simulink model "iir_butterworth"  (R2022b)
settings: Solver=VariableStepAuto  StartTime=0.0  StopTime=1  RelTol=1e-3
libraries: dspsrcs4 x3, simulink x1, dsparch4 x1
settings Model: Creator=HARIPREETA  LastModifiedBy=HARIPREETA

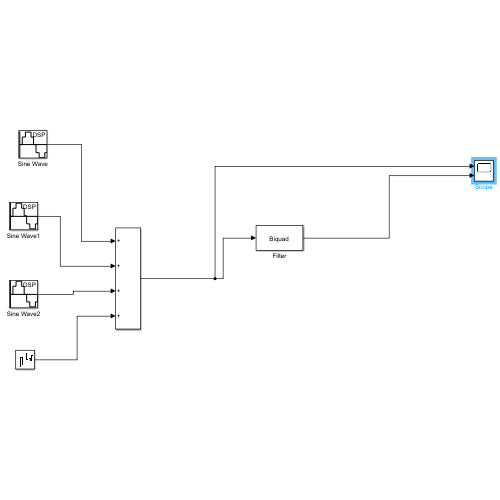
[thumbnail: Simulink's stored preview of the top-level diagram]
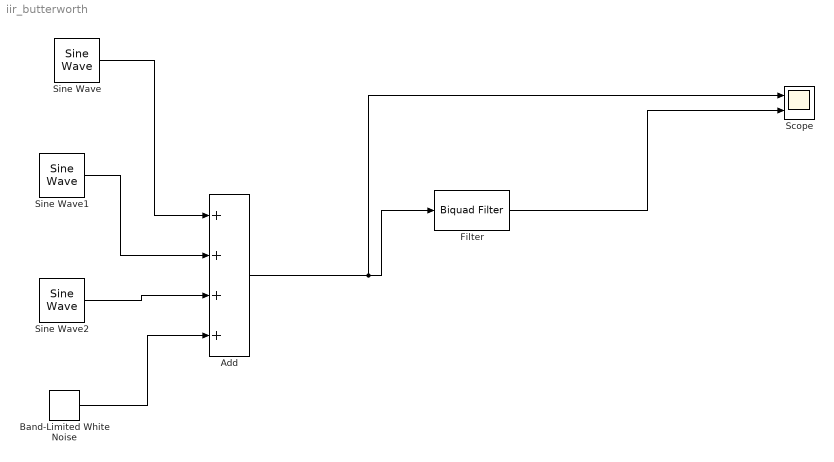
== system iir_butterworth ==
  Add : Sum  Inputs=++++
  Band-Limited White Noise : simulink/Sources/Band-Limited White Noise  Cov=[0.1]  Ts=1/1000  seed=[23341]
  Filter : dsparch4/Biquad Filter  Tag=BlockMethodSubSystem  FilterSource=Dialog parameters  CoeffSource=Specify via dialog  FilterObject=BQF  IIRFiltStruct=Direct form II  BiQuadCoeffs=[1 2 1 1 -1.85434463667763527 0.994401644019358599;1 2 1 1 -1.84402234363796702 0.983299717332608236;1 2 1 1 -1.83381787502916316 0.972324514251585392;1 2 1 1 -1.82373156100482814 0.961476389866104286;1 2 1 1 -1.81376367374963077 0.950755636918699909;1 2 1 1 -1.80391443006915608 0.940162488590091217;1 2 1 1 -1.79418399391444039 0.929697121214391187;1 2 1 1 -1.78457247884091474 0.919359656923772084;1 2 1 1 -1.77507995040165834 0.909150166222478573;1 2 1 1 -1.76570642847501214 0.899068670490245747;1 2 1 1 -1.75645188952676179 0.889115144415340453;1 2 1 1 -1.7473162688072239 0.879289518357593169;1 2 1 1 -1.73829946248369382 0.869591680641907172;1 2 1 1 -1.72940132970882798 0.860021479782863474;1 2 1 1 -1.72062169462562808 0.850578726641141314;1 2 1 1 -1.71196034830979404 0.841263196512572309;1 2 1 1 -1.70341705065028215 0.832074631150739208;1 2 1 1 -1.69499153216899412 0.823012740724101244;1 2 1 1 -1.68668349578056942 0.814077205708704232;1 2 1 1 -1.67849261849332576 0.805267678717589752;1 2 1 1 -1.67041855305242759 0.796583786268072913;1 2 1 1 -1.6624609295264241 0.788025130488107739;1 2 1 1 -1.65461935683831096 0.779591290762990496;1 2 1 1 -1.64689342424232277 0.771281825323691717;1 2 1 1 -1.63928270274767418 0.763096272778132634;1 2 1 1 -1.63178674649049427 0.755034153586738865;1 2 1 1 -1.62440509405520905 0.747094971483627024;1 2 1 1 -1.61713726974664485 0.739278214844788728;1 2 1 1 -1.60998278481412638 0.731583358004642914;1 2 1 1 -1.60294113862884657 0.724009862522332348;1 2 1 1 -1.5960118198157911 0.716557178399141237;1 2 1 1 -1.58919430734149114 0.709224745248404509;1 2 1 1 -1.58248807155887339 0.702011993419274338;1 2 1 1 -1.57589257521046955 0.694918345075701938;1 2 1 1 -1.5694072743912364 0.687943215231978544;1 2 1 1 -1.56303161947222424 0.681086012746166536;1 2 1 1 -1.55676505598631376 0.674346141272736621;1 2 1 1 -1.55060702547723084 0.667723000175706849;1 2 1 1 -1.54455696631302586 0.661215985403564299;1 2 1 1 -1.53861431446518893 0.654824490327225228;1 2 1 1 -1.53277850425454631 0.648547906542269459;1 2 1 1 -1.52704896906507082 0.642385624636663044;1 2 1 1 -1.52142514202670576 0.636337034925156475;1 2 1 1 -1.51590645666829249 0.630401528151526391;1 2 1 1 -1.51049234754165207 0.62457849615979355;1 2 1 1 -1.50518225081786383 0.618867332535538939;1 2 1 1 -1.49997560485674808 0.613267433218397384;1 2 1 1 -1.49487185075053897 0.607778197086795147;1 2 1 1 -1.48987043284271148 0.602399026515961555;1 2 1 1 -1.48497079922289488 0.597129327910225438;1 2 1 1 -1.48017240219879165 0.591968512210574671;1 2 1 1 -1.47547469874597703 0.586915995378430977;1 2 1 1 -1.47087715093645133 0.581971198856569782;1 2 1 1 -1.46637922634677831 0.577133550008084306;1 2 1 1 -1.46198039844661687 0.572402482534263068;1 2 1 1 -1.4576801469684415 0.567777436872235808;1 2 1 1 -1.45347795825921033 0.56325786057320093;1 2 1 1 -1.44937332561471877 0.558843208662034963;1 2 1 1 -1.44536574959736086 0.554532943979051618;1 2 1 1 -1.4414547383379841 0.550326537504657431;1 2 1 1 -1.43763980782251188 0.546223468667621059;1 2 1 1 -1.43392048216397772 0.542223225637655348;1 2 1 1 -1.43029629386059987 0.538325305602983306;1 2 1 1 -1.42676678404049606 0.534529215033535898;1 2 1 1 -1.42333150269362263 0.530834469930409392;1 2 1 1 -1.41999000889149585 0.527240596062182654;1 2 1 1 -1.41674187099524129 0.523747129188679383;1 2 1 1 -1.41358666685248591 0.52035361527273194;1 2 1 1 -1.41052398398359791 0.517059610680487558;1 2 1 1 -1.40755341975775372 0.513864682370772874;1 2 1 1 -1.40467458155929426 0.510768408074016245;1 2 1 1 -1.40188708694481856 0.507770376461205597;1 2 1 1 -1.39919056379143814 0.504870187303340323;1 2 1 1 -1.39658465043660107 0.502067451621816541;1 2 1 1 -1.39406899580988086 0.499361791830169044;1 2 1 1 -1.39164325955710155 0.496752841867573069;1 2 1 1 -1.38930711215716274 0.494240247324490956;1 2 1 1 -1.38706023503190146 0.491823665560833845;1 2 1 1 -1.38490232064932739 0.489502765816992536;1 2 1 1 -1.38283307262053512 0.487277229318070104;1 2 1 1 ...(+1136 chars)]  ScaleValues=[0.0350142518354308943;0.0348193434236603525;0.0346266598056056349;0.0344362072153190438;0.0342479907922672924;0.0340620146302338181;0.033878281824987741;0.0336967945207143418;0.0335175539552051011;0.0333405605038084099;0.0331658137221446658;0.0329933123875923232;0.032823054539553323;0.0326550375185089142;0.0324892580038782797;0.0323257120506945939;0.0321643951251142715;0.0320053021387768089;0.0318484274820337032;0.0316937650560660533;0.0315413083039113584;0.0313910502404209299;0.0312429834811698802;0.031097100270342265;0.0309533925076146202;0.0308118517740611636;0.0306724693571045273;0.0305352362745359776;0.030400143297629148;0.0302671809733714853;0.0301363396458375621;0.0300076094767283211;0.0298809804651002202;0.0297564424663081285;0.0296339852101855546;0.0295135983184856045;0.0293952713216057183;0.0292789936746190096;0.0291647547726346032;0.0290525439655090964;0.0289423505719308;0.0288341638928980952;0.0287279732246127108;0.0286237678708084718;0.028521537154535398;0.0284212704294187872;0.0283229570904123575;0.0282265865840640381;0.0281321484183125678;0.0280396321718326402;0.0279490275029457662;0.0278603241581135246;0.027773511980029638;0.0276885809153264995;0.0276055210219115776;0.0275243224759485761;0.027444975578497708;0.0273674707618290769;0.0272917985954227206;0.0272179497916683263;0.0271459152112773043;0.0270756858684194288;0.0270072529355958706;0.0269406077482599454;0.0268757418091967008;0.0268126467926717155;0.0267513145483595505;0.0266917371050615394;0.0266339066742224059;0.0265778156532548125;0.0265234566286805459;0.0264708223790968041;0.0264199058779755816;0.0263707002963038534;0.0263231990050720524;0.0262773955776178549;0.0262332837918320683;0.0261908576322331041;0.0261501112919162795;0.0261110391743837426;0.0260736358952607349;0.0260378962839035409;0.0260038153849041428;0.0259713884594964979;0.0259406109868689297;0.0259114786653870458;0.0258839874137311958;0.0258581333719523423;0.0258339129024499972;0.0258113225908755441;0.0257903592469641493;0.0257710199052982661;0.0257533018260053086;0.0257372024953922453;0.0257227196265191714;0.0257098511597141921;0.0256985952630314173;0.0256889503326537538;0.0256809149932421231;0.0256744880982322822;0.02566966873008052;0.0256664562004590424;0.025664850050401887;1]  IC=0  ICnum=0  ICden=0  a0Flag=Warning  optimizeScaleValues=on  ScaleValueMode=Specify via input port (g)  InputProcessing=Columns as channels (frame based)  roundingMode=Floor  overflowMode=off  scaleValueFracLength=14  denProdOutputFracLength=30  denAccumFracLength=30  secondMemoryFracLength=15
  Scope : Scope  NumInputPorts=2
  Sine Wave : dspsrcs4/Sine Wave  Amplitude=150  Frequency=50  Phase=0  SampleMode=Discrete  OutComplex=Real  CompMethod=Trigonometric fcn  TableSize=Speed  SampleTime=1/1000  SamplesPerFrame=1  ResetState=Restart at time zero  OutputFrames=off  dataType=double  wordLen=16  udDataType=sfix(16)  fracBitsMode=Best precision  numFracBits=15  OutDataTypeStr=double  LastOutDataTypeStr=double
  Sine Wave1 : dspsrcs4/Sine Wave  Amplitude=20  Frequency=150  Phase=0  SampleMode=Discrete  OutComplex=Real  CompMethod=Trigonometric fcn  TableSize=Speed  SampleTime=1/1000  SamplesPerFrame=1  ResetState=Restart at time zero  OutputFrames=off  dataType=double  wordLen=16  udDataType=sfix(16)  fracBitsMode=Best precision  numFracBits=15  OutDataTypeStr=double  LastOutDataTypeStr=double
  Sine Wave2 : dspsrcs4/Sine Wave  Amplitude=3  Frequency=250  Phase=0  SampleMode=Discrete  OutComplex=Real  CompMethod=Trigonometric fcn  TableSize=Speed  SampleTime=1/1000  SamplesPerFrame=1  ResetState=Restart at time zero  OutputFrames=off  dataType=double  wordLen=16  udDataType=sfix(16)  fracBitsMode=Best precision  numFracBits=15  OutDataTypeStr=double  LastOutDataTypeStr=double
  wires:
  Filter/1 -> Scope/2
  Add/1 -> Scope/1, Filter/1
  Sine Wave/1 -> Add/1
  Sine Wave1/1 -> Add/2
  Sine Wave2/1 -> Add/3
  Band-Limited White Noise/1 -> Add/4
